simulink model "FP667_Jerrar_Bukhari_Luenberger_Linear"  (R2017b)
settings: Solver=FixedStepAuto  StartTime=0.0  StopTime=60  FixedStep=0.05  RelTol=1e-3
values from neighbouring files (symbols this model uses):
  A = [0 1 0 0 0 0 ... (first row only)    [ENPM667FinalProject_JerrarBukhari_MatlabCode.m]
  B = [ 0 ... (first row only)    [ENPM667FinalProject_JerrarBukhari_MatlabCode.m]
  C = [ 1 0 0 0 0 0 ... (first row only)    [ENPM667FinalProject_JerrarBukhari_MatlabCode.m]
  L = place(A',C',P)'    [ENPM667FinalProject_JerrarBukhari_MatlabCode.m]
undefined symbols (not defined in the file or in its folder): K
settings Model: Creator=Jerrar  LastModifiedBy=Jerrar

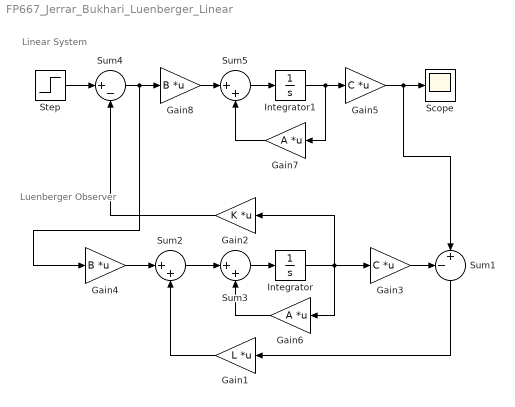
== system FP667_Jerrar_Bukhari_Luenberger_Linear ==
  note: Linear System
  note: Luenberger
      |  Observer
  Gain1 : Gain  Gain=L  Multiplication=Matrix(K*u)
  Gain2 : Gain  Gain=K  Multiplication=Matrix(K*u)
  Gain3 : Gain  Gain=C  Multiplication=Matrix(K*u)
  Gain4 : Gain  Gain=B  Multiplication=Matrix(K*u)
  Gain5 : Gain  Gain=C  Multiplication=Matrix(K*u)
  Gain6 : Gain  Gain=A  Multiplication=Matrix(K*u)
  Gain7 : Gain  Gain=A  Multiplication=Matrix(K*u)
  Gain8 : Gain  Gain=B  Multiplication=Matrix(K*u)
  Integrator : Integrator
  Integrator1 : Integrator
  Scope : Scope
  Step : Step  SampleTime=0
  Sum1 : Sum  Inputs=-+|
  Sum2 : Sum  Inputs=|++
  Sum3 : Sum  Inputs=|++
  Sum4 : Sum  Inputs=|+-
  Sum5 : Sum  Inputs=|++
  wires:
  Gain1/1 -> Sum2/2
  Gain4/1 -> Sum2/1
  Integrator/1 -> Gain2/1, Gain6/1, Gain3/1
  Sum2/1 -> Sum3/1
  Gain6/1 -> Sum3/2
  Sum3/1 -> Integrator/1
  Gain2/1 -> Sum4/2
  Step/1 -> Sum4/1
  Gain3/1 -> Sum1/1
  Sum1/1 -> Gain1/1
  Integrator1/1 -> Gain5/1, Gain7/1
  Sum5/1 -> Integrator1/1
  Sum4/1 -> Gain8/1, Gain4/1
  Gain7/1 -> Sum5/2
  Gain8/1 -> Sum5/1
  Gain5/1 -> Scope/1, Sum1/2
